simulink model "Motor1"  (R2018a)
settings: Solver=FixedStepAuto  StartTime=0.0  StopTime=10  RelTol=1e-3  EnableMultiTasking=on
libraries: legoev3lib x2, simulink_extras x1
settings Model: SimulationMode=external  ExtModeTrigDuration=2  Creator=Lenovo  LastModifiedBy=Lenovo
settings SolverCC: PositivePriorityOrder=on
settings OptimizationCC: EnhancedBackFolding=on  PassReuseOutputArgsThreshold=0  MaxStackSize=64  OptimizeBlockOrder=speed  DifferentSizesBufferReuse=on  OptimizationCustomize=off
settings DebuggingCC: ParameterTunabilityLossMsg=error
settings HardwareCC: ProdBitPerPointer=32  ProdBitPerSizeT=32  ProdBitPerPtrDiffT=32  ProdLargestAtomicInteger=Long  ProdWordSize=32  ProdHWDeviceType=ARM Compatible->ARM 9  UseEmbeddedCoderFeatures=off  UseSimulinkCoderFeatures=off
settings SFSimCC: MATLABDynamicMemAlloc=off
settings RTWCC: SystemTargetFile=ert.tlc  HardwareBoard=LEGO MINDSTORMS EV3  TLCOptions="-aInlineSetEventsForThisBaseRateFcn=TLC_FALSE -aSuppressMultiTaskScheduler=TLC_FALSE  -aRateBasedStepFcn=0"  TemplateMakefile=ert_default_tmf  GenerateReport=on  Toolchain=Sourcery G++ Lite v2009q3  LaunchReport=on
settings CodeAppCC: ForceParamTrailComments=on  OperatorAnnotations=on
settings ERTTargetCC: ERTCustomFileBanners=off  SupportContinuousTime=on  SupportNonInlinedSFcns=on  RemoveResetFunc=off  SupportVariableSizeSignals=on  ModelStepFunctionPrototypeControlCompliant=off

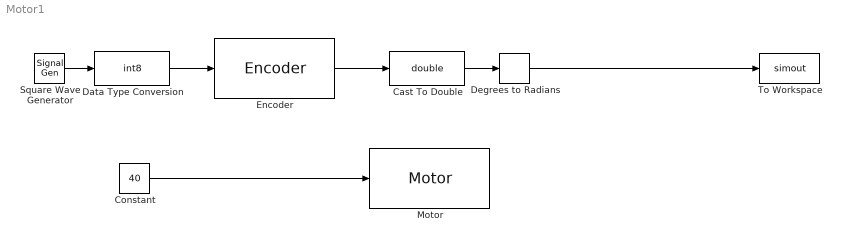
== system Motor1 ==
  Cast To Double : DataTypeConversion  OutDataTypeStr=double
  Constant : Constant  Value=40
  Data Type Conversion : DataTypeConversion  OutDataTypeStr=int8
  Degrees to Radians : simulink_extras/Transformations/Degrees to Radians
  Encoder : legoev3lib/Encoder  portNumber=A  opMode=Reset by external signal  sampleTime=0.1
      settings: SourceProductName=Simulink Support Package for LEGO MINDSTORMS EV3 Hardware  SourceProductBaseCode=LEGOEV3
  Motor : legoev3lib/Motor  sportNumber=A  sstopAction=Brake
  Square Wave Generator : SignalGenerator  WaveForm=square  Units=rad/sec
  To Workspace : ToWorkspace  VariableName=simout  SaveFormat=Structure With Time  SampleTime=-1
  wires:
  Constant/1 -> Motor/1
  Encoder/1 -> Cast To Double/1
  Degrees to Radians/1 -> To Workspace/1
  Cast To Double/1 -> Degrees to Radians/1
  Square Wave Generator/1 -> Data Type Conversion/1
  Data Type Conversion/1 -> Encoder/1
